simulink model "communication2"  (R2025b)
settings: Solver=FixedStepAuto  StartTime=0.0  StopTime=100  FixedStep=0.01  RelTol=1e-3
undefined symbols (not defined in the file or in its folder): aruco_markers, f, LF, T_sidewc, T_topwc, u_offset
libraries: instrumentseriallib x4, instrumentlib x2
settings Model: ExtModeTrigDuration=2  Creator=CoolA  LastModifiedBy=CoolA
settings SolverCC: AutoInsertRateTranBlk=on
settings OptimizationCC: EnhancedBackFolding=on  PassReuseOutputArgsAs=Individual arguments  ZeroExternalMemoryAtStartup=off  ZeroInternalMemoryAtStartup=off  MaxStackSize=64  OptimizeBlockOrder=speed  DifferentSizesBufferReuse=on  OptimizationCustomize=off  EfficientTunableParamExpr=on
settings DebuggingCC: ParameterTunabilityLossMsg=error
settings HardwareCC: ProdBitPerInt=16.0  ProdBitPerPointer=16.0  ProdBitPerSizeT=16.0  ProdBitPerPtrDiffT=16.0  ProdLargestAtomicFloat=None  ProdWordSize=8.0  ProdHWDeviceType=Atmel->AVR  UseEmbeddedCoderFeatures=off  UseSimulinkCoderFeatures=off
settings RTWCC: SystemTargetFile=ert.tlc  HardwareBoard=Arduino Uno  TemplateMakefile=ert_default_tmf  Toolchain=Arduino AVR  Description=Embedded Coder
settings CodeAppCC: ForceParamTrailComments=on  IgnoreCustomStorageClasses=off  OperatorAnnotations=on  SimulinkDataObjDesc=on  SFDataObjDesc=on  InsertBlockDesc=on
settings ERTTargetCC: ExtModeTransport=3.0  ExtModeStaticAlloc=on  ExtModeAutomaticAllocSize=off  ExtModeStaticAllocSize=250.0  ExtModeMexFile=ext_xcp  ExtModeIntrfLevel=Level2 - Open  InlinedParameterPlacement=Hierarchical  SupportContinuousTime=on  SupportNonInlinedSFcns=on  SupportVariableSizeSignals=on

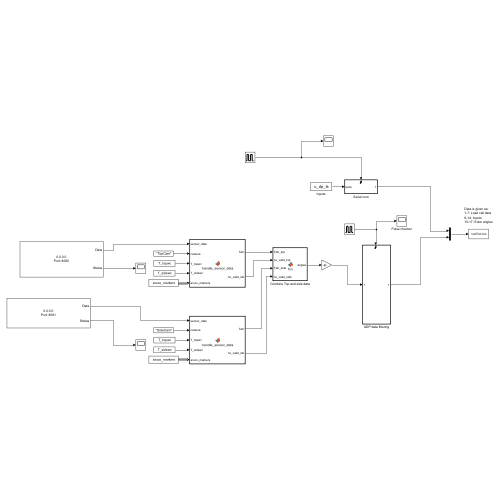
[thumbnail: Simulink's stored preview of the top-level diagram]
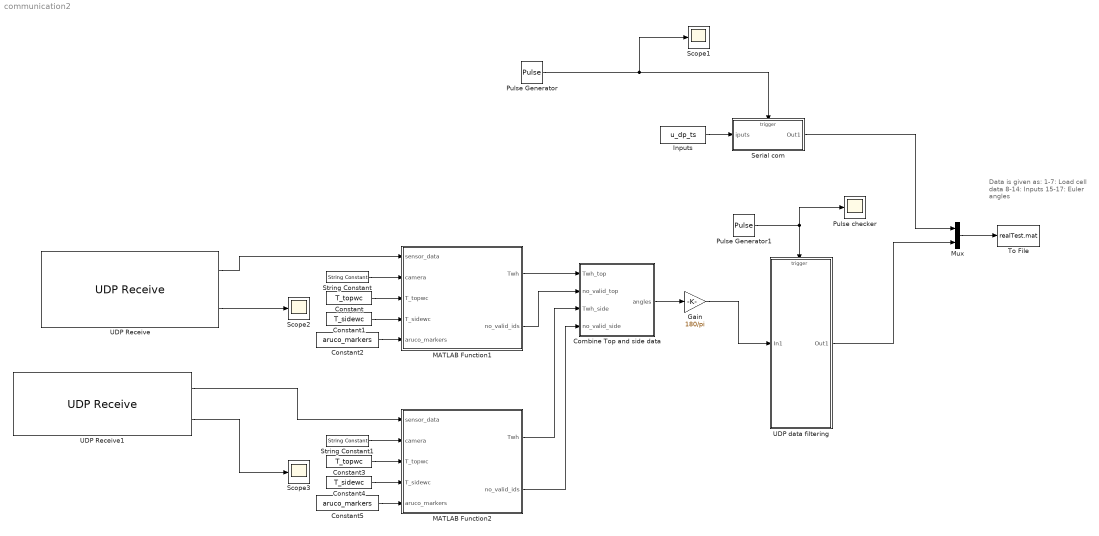
== system communication2 ==
  note: Data is given as:
      | 1-7: Load cell data
      | 8-14: Inputs
      | 15-17: Euler angles
  Combine Top and side data : MATLAB Function  TreatAsAtomicUnit=on
  Constant : Constant  Value=T_topwc
  Constant1 : Constant  Value=T_sidewc
  Constant2 : Constant  Value=aruco_markers  OutDataTypeStr=Bus: aruco_marker_bus
  Constant3 : Constant  Value=T_topwc
  Constant4 : Constant  Value=T_sidewc
  Constant5 : Constant  Value=aruco_markers  OutDataTypeStr=Bus: aruco_marker_bus
  Gain : Gain  Gain=180/pi
  Inputs : FromWorkspace  VariableName=u_dp_ts  SampleTime=-1
  MATLAB Function1 : MATLAB Function  TreatAsAtomicUnit=on
  MATLAB Function2 : MATLAB Function  TreatAsAtomicUnit=on
  Mux : Mux  Inputs=2
  Pulse Generator : DiscretePulseGenerator  PulseType=Time based  Period=0.02  PulseWidth=50
  Pulse Generator1 : DiscretePulseGenerator  PulseType=Time based  Period=0.1  PulseWidth=10
  Pulse checker : Scope
      settings: ActiveDisplayYMinimum=-0.12499999999999997  ActiveDisplayYMaximum=1.125  DataLoggingVariableName=ScopeData5
  Scope1 : Scope
      settings: ActiveDisplayYMinimum=-1  ActiveDisplayYMaximum=1
  Scope2 : Scope
      settings: ActiveDisplayYMinimum=-0.12499999999999997  ActiveDisplayYMaximum=1.125  DataLoggingVariableName=ScopeData8
  Scope3 : Scope
      settings: ActiveDisplayYMinimum=-0.12499999999999997  ActiveDisplayYMaximum=1.125
  Serial com : Subsystem  TreatAsAtomicUnit=on
  String Constant : StringConstant  String="\"TopCam\""
  String Constant1 : StringConstant  String="\"SideCam\""
  To File : ToFile  Filename=realTest.mat  SaveFormat=Timeseries
  UDP Receive : instrumentlib/UDP Receive  LocalAddress=0.0.0.0  LocalPort=8080  EnablePortSharing=off  Host=localhost  Port=9090  GetLatestData=on  DataSize=[ 350, 1 ]  DataType=uint8  ASCIIFormatting=%f,  Terminator=LF  CustomTerminator=10  ByteOrder=big-endian  EnableBlockingMode=off  Timeout=10  SampleTime=0.01  SimulateUsing=Interpreted execution
  UDP Receive1 : instrumentlib/UDP Receive  LocalAddress=0.0.0.0  LocalPort=8081  EnablePortSharing=off  Host=localhost  Port=9090  GetLatestData=on  DataSize=[ 350, 1 ]  DataType=uint8  ASCIIFormatting=%f,  Terminator=LF  CustomTerminator=10  ByteOrder=big-endian  EnableBlockingMode=off  Timeout=10  SampleTime=0.01  SimulateUsing=Interpreted execution
  UDP data filtering : Subsystem
  wires:
  Pulse Generator/1 -> Serial com/Trigger, Scope1/1
  MATLAB Function1/2(no_valid_ids) -> Combine Top and side data/2(no_valid_top)
  String Constant1/1 -> MATLAB Function2/2(camera)
  Constant/1 -> MATLAB Function1/3(T_topwc)
  UDP Receive1/2 -> Scope3/1
  Pulse Generator1/1 -> UDP data filtering/Trigger, Pulse checker/1
  UDP Receive/2 -> Scope2/1
  String Constant/1 -> MATLAB Function1/2(camera)
  Constant3/1 -> MATLAB Function2/3(T_topwc)
  Constant4/1 -> MATLAB Function2/4(T_sidewc)
  MATLAB Function1/1(Twh) -> Combine Top and side data/1(Twh_top)
  Gain/1 -> UDP data filtering/1(In1)
  UDP Receive/1 -> MATLAB Function1/1(sensor_data)
  UDP Receive1/1 -> MATLAB Function2/1(sensor_data)
  Constant5/1 -> MATLAB Function2/5(aruco_markers)
  MATLAB Function2/1(Twh) -> Combine Top and side data/3(Twh_side)
  Combine Top and side data/1(angles) -> Gain/1
  Constant2/1 -> MATLAB Function1/5(aruco_markers)
  MATLAB Function2/2(no_valid_ids) -> Combine Top and side data/4(no_valid_side)
  Constant1/1 -> MATLAB Function1/4(T_sidewc)
  Serial com/1(Out1) -> Mux/1
  UDP data filtering/1(Out1) -> Mux/2
  Mux/1 -> To File/1
  Inputs/1 -> Serial com/1(iputs)

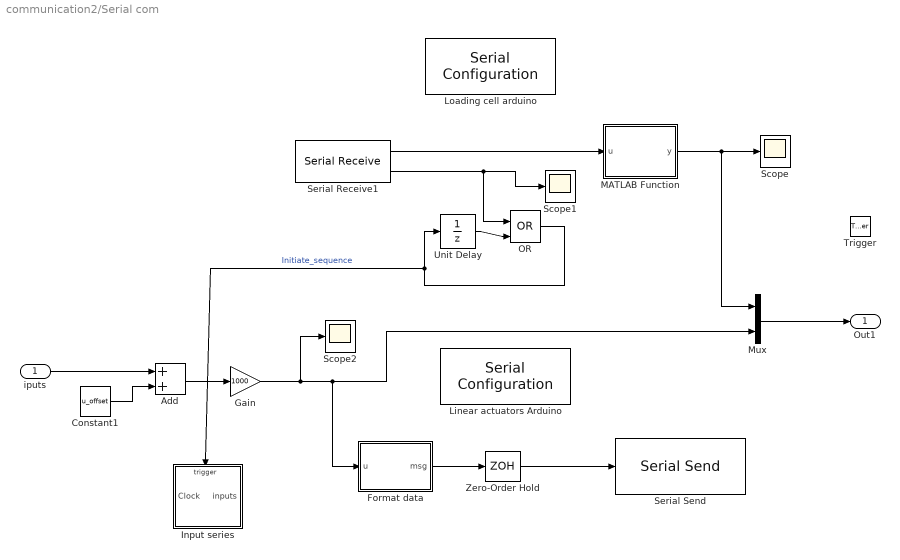
== system communication2/Serial com ==
  iputs : Inport
  Trigger : TriggerPort  VariantControl=(inherit)
  Add : Sum
  Constant1 : Constant  Value=u_offset
  Format data : MATLAB Function  TreatAsAtomicUnit=on
  Gain : Gain  Gain=1000
  Input series : Subsystem
  Linear actuators Arduino : instrumentseriallib/Serial Configuration  Priority=-200000  PortSel=COM3  Port=COM3  ComPort=COM3  BaudRate=115200  DataBits=8  Parity=none  StopBits=1  ByteOrder=little-endian  FlowControl=none  Timeout=10  SimulateUsing=Interpreted execution  BlockInModel=on  aMode=1
  Loading cell arduino : instrumentseriallib/Serial Configuration  Priority=-200000  PortSel=COM6  Port=COM6  ComPort=COM6  BaudRate=460800  DataBits=8  Parity=none  StopBits=1  ByteOrder=little-endian  FlowControl=none  Timeout=10  SimulateUsing=Interpreted execution  BlockInModel=on  aMode=1
  MATLAB Function : MATLAB Function  TreatAsAtomicUnit=on
  Mux : Mux  Inputs=2
  OR : Logic  Operator=OR  IconShape=distinctive  AllPortsSameDT=off  OutDataTypeStr=boolean
  Scope : Scope
      settings: ActiveDisplayYMinimum=-3015.125  ActiveDisplayYMaximum=2906.125  DataLoggingVariableName=ScopeData6
  Scope1 : Scope
      settings: ActiveDisplayYMinimum=-0.12499999999999997  ActiveDisplayYMaximum=1.125  DataLoggingVariableName=ScopeData7
  Scope2 : Scope
      settings: ActiveDisplayYMinimum=57.934587069134736  ActiveDisplayYMaximum=122.86701751523671  DataLoggingVariableName=ScopeData9
  Serial Receive1 : instrumentseriallib/Serial Receive  Priority=1  PortSel=COM6  Port=COM6  ComPort=COM6  DataType=uint8  SaveDataType=uint8  ToggleHeader=off  Header=[]  ToggleDataSize=on  DataSize=[15 1]  ToggleTerminator=off  Terminator=<none>  CustomTerminator=[]  InputFormat=Column major  EnableBlockingMode=off  ActionDataUnavailable=Output last received value  ActionWhenDataUnavailable=Output last received value  CustomValue=0  SampleTime=-1  SimulateUsing=Interpreted execution  BlockInModel=on  aMode=1  LibraryInUse=instrumentlib
  Serial Send : instrumentseriallib/Serial Send  Priority=1  PortSel=COM3  Port=COM3  ComPort=COM3  Header=[]  Terminator=LF ('\n')  CustomTerminator=[]  EnableBlockingMode=on  SimulateUsing=Interpreted execution  BlockInModel=on  aMode=1
  Unit Delay : UnitDelay  SampleTime=-1  HasFrameUpgradeWarning=on
  Zero-Order Hold : ZeroOrderHold  SampleTime=-1
  Out1 : Outport
  wires:
  Zero-Order Hold/1 -> Serial Send/1
  Format data/1(msg) -> Zero-Order Hold/1
  Serial Receive1/1 -> MATLAB Function/1(u)
  MATLAB Function/1(y) -> Mux/1, Scope/1
  Serial Receive1/2 -> OR/1, Scope1/1
  OR/1 -> Input series/Trigger, Unit Delay/1  "Initiate_sequence"
  Unit Delay/1 -> OR/2
  Mux/1 -> Out1/1
  Add/1 -> Gain/1
  iputs/1 -> Add/1
  Constant1/1 -> Add/2
  Gain/1 -> Format data/1(u), Mux/2, Scope2/1

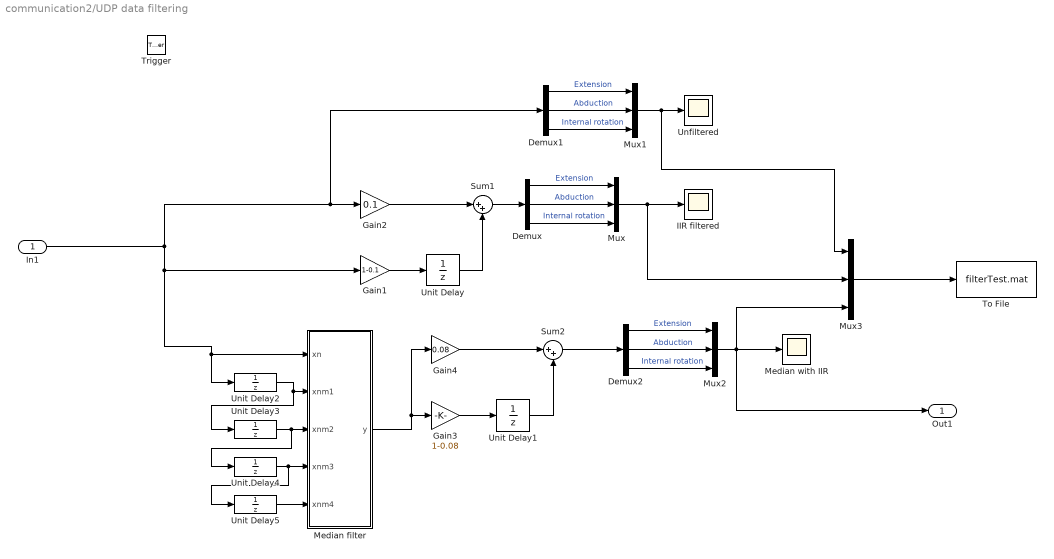
== system communication2/UDP data filtering ==
  In1 : Inport
  Trigger : TriggerPort  VariantControl=(inherit)  PortDimensions=1
  Demux : Demux  Outputs=3
  Demux1 : Demux  Outputs=3
  Demux2 : Demux  Outputs=3
  Gain1 : Gain  Gain=1-0.1
  Gain2 : Gain  Gain=0.1
  Gain3 : Gain  Gain=1-0.08
  Gain4 : Gain  Gain=0.08
  IIR filtered : Scope
      settings: ActiveDisplayYMinimum=-72.522527102781169  ActiveDisplayYMaximum=75.739145629510645  DataLoggingVariableName=ScopeData2
  Median filter : MATLAB Function  TreatAsAtomicUnit=on
  Median with IIR : Scope
      settings: ActiveDisplayYMinimum=-69.815239088721853  ActiveDisplayYMaximum=74.872619576986168  DataLoggingVariableName=ScopeData3
  Mux{,1..3} (4 alike) : Mux  Inputs=3
  Sum1 : Sum  Inputs=|++
  Sum2 : Sum  Inputs=|++
  To File : ToFile  Filename=filterTest.mat  SaveFormat=Timeseries
  Unfiltered : Scope
      settings: ActiveDisplayYMinimum=-89.516578788541381  ActiveDisplayYMaximum=94.920329470501926  DataLoggingVariableName=ScopeData4
  Unit Delay{,1..5} (6 alike) : UnitDelay  InitialCondition=zeros(3,1)  SampleTime=-1  HasFrameUpgradeWarning=on
  Out1 : Outport
  wires:
  Sum2/1 -> Demux2/1
  Unit Delay1/1 -> Sum2/2
  Demux/3 -> Mux/3  "Internal rotation"
  Gain4/1 -> Sum2/1
  Demux2/3 -> Mux2/3  "Internal rotation"
  Unit Delay/1 -> Sum1/2
  Gain1/1 -> Unit Delay/1
  Unit Delay3/1 -> Unit Delay4/1, Median filter/3(xnm2)
  Mux2/1 -> Out1/1, Mux3/3, Median with IIR/1
  Demux2/2 -> Mux2/2  "Abduction"
  In1/1 -> Gain1/1, Unit Delay2/1, Median filter/1(xn), Demux1/1, Gain2/1
  Gain2/1 -> Sum1/1
  Mux1/1 -> Mux3/1, Unfiltered/1
  Unit Delay2/1 -> Unit Delay3/1, Median filter/2(xnm1)
  Demux1/3 -> Mux1/3  "Internal rotation"
  Demux1/1 -> Mux1/1  "Extension"
  Median filter/1(y) -> Gain4/1, Gain3/1
  Demux/1 -> Mux/1  "Extension"
  Demux2/1 -> Mux2/1  "Extension"
  Demux/2 -> Mux/2  "Abduction"
  Sum1/1 -> Demux/1
  Demux1/2 -> Mux1/2  "Abduction"
  Mux/1 -> Mux3/2, IIR filtered/1
  Gain3/1 -> Unit Delay1/1
  Unit Delay5/1 -> Median filter/5(xnm4)
  Unit Delay4/1 -> Unit Delay5/1, Median filter/4(xnm3)
  Mux3/1 -> To File/1

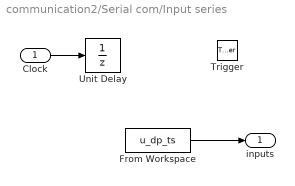
== system communication2/Serial com/Input series ==
  Clock : Inport
  Trigger : TriggerPort  VariantControl=(inherit)  PortDimensions=1
  From Workspace : FromWorkspace  VariableName=u_dp_ts  SampleTime=-1
  Unit Delay : UnitDelay  SampleTime=-1  HasFrameUpgradeWarning=on
  inputs : Outport
  wires:
  From Workspace/1 -> inputs/1
  Clock/1 -> Unit Delay/1

== matlab function communication2/Serial com/MATLAB Function ==
  data: u input; y output size=[7 1]
function y = parseSerial(u)

persistent buffer
persistent previous_output

if isempty(previous_output)
    previous_output = zeros(7,1);
end

if isempty(buffer)
    buffer = '';
end

% Append new data
buffer = [buffer char(u')];

y = previous_output;  % default output

while true
    
    startIdx = strfind(buffer, '<');
    endIdx   = strfind(buffer, '>');
    
    % Need both markers
    if isempty(startIdx) || isempty(endIdx)
        y = previous_output;
        break;
    end
    
    % Case 1: end comes before start → discard garbage
    if endIdx(1) < startIdx(1)
        buffer = buffer(endIdx(1)+1:end);
        continue;
    end
    
    % Case 2: valid packet exists
    if startIdx(1) < endIdx(1)
        
        msg = buffer(startIdx(1)+1 : endIdx(1)-1);
        %disp(msg)
        
        % Remove processed part
        buffer = buffer(endIdx(1)+1:end);
        
        vals = sscanf(msg, '%f,%f,%f,%f,%f,%f,%f');
        
        if numel(vals) == 7 && all(abs(vals) < 10000)
            y = zeros(7,1);
            y(:) = vals(1:7);  
            previous_output = y;
            return;   % exit after one valid packet
        end
    end
end

== matlab function communication2/Serial com/Format data ==
  data: u input; msg output uint8 size=[1 29]
% function msg = fcn(u)
% MAX_LEN = 30;
% u = int8(u);
% msg = sprintf('<%03d,%03d,%03d,%03d,%03d,%03d,%03d>\n', u(1), u(2), u(3), u(4), u(5), u(6), u(7));
% 
% % 03 ensures 3 digits

function msg = formatData(u)
%#codegen

MAX_LEN = 29;
msg = uint8(zeros(1, MAX_LEN));

u = int16(u);

str = sprintf('<%03d,%03d,%03d,%03d,%03d,%03d,%03d>', ...
    u(1), u(2), u(3), u(4), u(5), u(6), u(7));

len = min(length(str), MAX_LEN);
msg(1:len) = uint8(str(1:len));

== matlab function communication2/Combine Top and side data ==
  data: Twh_top input; no_valid_top input; angles output; Twh_side input; no_valid_side input
function angles = fcn(Twh_top, no_valid_top, Twh_side, no_valid_side)
Twhs = [];
if ~no_valid_top
    Twhs = Twh_top;
end
if ~no_valid_side
    Twhs = [Twhs, Twh_side];
end

if isempty(Twhs)
    disp("No valid ids detected")
    angles = zeros(3,1);
else
    Twh = average_translations(Twhs);
    angles = tranmat2euler(Twh);
end

== matlab function communication2/MATLAB Function1 ==
  data: sensor_data input; Twh output; camera input; T_topwc input; T_sidewc input; aruco_markers input; no_valid_ids output
function [Twh, no_valid_ids] = handle_sensor_data(sensor_data, camera, T_topwc, T_sidewc, aruco_markers)
%angles = zeros(3,1);
Twh = zeros(4,4);
handle_successful = false;
[IDs, rvecs, tvecs] = parse_sensor_data(sensor_data);
%disp(sensor_data)
%disp(IDs)
%disp(rvecs)
%disp(tvecs)
% Legg til handle_successful i parse_sensor_data

[Twhs, no_valid_ids] = meas2Twh(IDs, rvecs, tvecs, camera, T_topwc, T_sidewc, aruco_markers);


if no_valid_ids
    disp("No valid ids detected")
else
    Twh = average_translations(Twhs);
    %[angles] = tranmat2euler(Twh);
end

== matlab function communication2/MATLAB Function2 ==
  data: sensor_data input; Twh output; camera input; T_topwc input; T_sidewc input; aruco_markers input; no_valid_ids output
function [Twh, no_valid_ids] = handle_sensor_data(sensor_data, camera, T_topwc, T_sidewc, aruco_markers)
%angles = zeros(3,1);
%handle_successful = false;
[IDs, rvecs, tvecs] = parse_sensor_data(sensor_data);
%disp(sensor_data)
%disp(IDs)
%disp(rvecs)
%disp(tvecs)
% Legg til handle_successful i parse_sensor_data

[Twhs, no_valid_ids] = meas2Twh(IDs, rvecs, tvecs, camera, T_topwc, T_sidewc, aruco_markers);


if no_valid_ids
    disp("No valid ids detected")
    Twh = zeros(4,4);
else
    Twh = average_translations(Twhs);
    %[angles] = tranmat2euler(Twh);
end

== matlab function communication2/UDP data filtering/Median filter ==
  data: xn input; y output; xnm1 input; xnm2 input; xnm3 input; xnm4 input
function y = fcn(xn,xnm1, xnm2, xnm3, xnm4)
x = [xn, xnm1, xnm2, xnm3, xnm4]';
y = median(x)';
